simulink model "SF049A_LoaMgr"  (R2013b)
settings: Solver=FixedStepDiscrete  SolverMode=SingleTasking  StartTime=0.0  StopTime=1  FixedStep=0.002  RelTol=1e-3
undefined symbols (not defined in the file): CURRMEASLOAMTGTNMASK_CNT_U08, IVTRLOAMTGTNMASK_CNT_U08, LoaCtrldShtdwn, LoaCurrMeasIdptSigNrFlt, LoaHwTqIdptSigNrFlt, LoaImdtShtdwn, LoaIvtrIdptSigNrFlt, LOAMAXSLEW_ULSPERSEC_F32, LoaMgrCurrIvtrMtgtnRate, LoaMgrCurrIvtrMtgtnSca, LoaMgrCurrIvtrMtgtnScaZeroEna, LoaMgrCurrMeasIdptSig0Resp, LoaMgrCurrMeasIdptSig1Resp, LoaMgrCurrMeasIdptSig2Resp, LoaMgrCurrMeasIdptSigFltThd, LoaMgrCurrMeasMtgtnRate, LoaMgrCurrMeasMtgtnSca, LoaMgrCurrMeasMtgtnScaZeroEna, LoaMgrFadeOutStRate, LoaMgrHwTqIdptSig0NoTqLoaResp, LoaMgrHwTqIdptSig1NoTqLoaResp, LoaMgrHwTqIdptSig2Resp, LoaMgrHwTqIdptSig4Resp, LoaMgrHwTqIdptSigFltThd, LoaMgrHwTqLoaAvlResp, LoaMgrIvtrIdptSig0Resp, LoaMgrIvtrIdptSig1Resp, LoaMgrIvtrIdptSig2Resp, LoaMgrIvtrIdptSigFltThd, LoaMgrIvtrMtgtnRate, LoaMgrIvtrMtgtnSca, LoaMgrIvtrMtgtnScaZeroEna, LoaMgrLimdStRate, LoaMgrLimdStSca, LoaMgrMotAgAvlSnsrlsResp, LoaMgrMotAgIdptSig0NoSnsrlsResp, LoaMgrMotAgIdptSig1NoSnsrlsResp, LoaMgrMotAgIdptSig2Resp, LoaMgrMotAgIdptSig3Resp, LoaMgrMotAgIdptSigFltThd, LoaMgrMotAgMtgtnRate, LoaMgrMotAgMtgtnSca, LoaMgrMotAgMtgtnScaZeroEna, LoaMotAgIdptSigNrFlt, LOASCAONE_ULS_F32, LOASCAZERO_ULS_F32, LoaSt1, LOASTIMDTSHTDWN_CNT_U08, LOASTNORM_CNT_U08, LOASTSWMTGTN_CNT_U08, MAXCURRMEASIDPTSIGALLWD_CNT_U08, MAXHWTQIDPTSIGALLWD_CNT_U08, MAXIVTRIDPTSIGALLWD_CNT_U08, MAXMOTAGMECLIDPTSIGALLWD_CNT_U08, NODEBSTEP_CNT_U16, NtcSts1, SigQlfr1
libraries: simulink x30, NxtrMin x4, NxtrMax x4, NxtrLim x2
(part 2 of 7)

== system SF049A_LoaMgr/ISO Fault Debounce/DiagMgr/NTCSTS_PREFAILD ==
  EA : Inport
  DS : Inport  Port=2
  TS : Inport  Port=3
  Qlf : Inport  Port=4
  Action Port : ActionPort  ActionType=case
  CopyRight2 : Subsystem  Description=|  mask(Copyright Information){none=on}
      | Copyright info block.                                               
      |                                                                     
      | Place copyright information at the top of every subsystem in design.
      mask prompts: none "No parameters"
      mask help: Place copyright information at the top of every subsystem in design.
      mask Display:
      | NxtrConf = 'Nexteer Confidential';
      | 
      | sys = bdroot; %handle for the current model ("system")
      | first = get_param(sys,'Created');
      | first = first(end-3:end);  %year is last four digits
      | 
      | last = get_param(sys,'LastModifiedDate');
      | if isempty(last)
      |     last = datestr(now,'yyyy');
      | else
      |     last = last(end-3:end);
      | end
      | 
      | if strcmp(first,last)
      |     fprintf('%s -- Copyright %s Nexteer',NxtrConf,first)
      | else
      |     fprintf('%s -- %s%s- %s Nexteer',NxtrConf,char(169),first,last)
      | end
  Data Type Conversion : DataTypeConversion
  If : If  IfExpression=u1 <= 0
  If Action Subsystem : Subsystem  TreatAsAtomicUnit=on
  If Action Subsystem1 : Subsystem  TreatAsAtomicUnit=on
  Merge : Merge
  Merge1 : Merge
  EAo : Outport
  Qlfo : Outport  Port=2
  wires:
  EA/1 -> If Action Subsystem1/2(EA), If/1
  If/1 -> If Action Subsystem/Action
  If/2 -> If Action Subsystem1/Action
  DS/1 -> Data Type Conversion/1, If Action Subsystem1/1(DS)
  TS/1 -> If Action Subsystem1/4(TS)
  If Action Subsystem/1(EAo) -> Merge/1
  If Action Subsystem1/1(EAo) -> Merge/2
  If Action Subsystem1/2(Qlfo) -> Merge1/2
  If Action Subsystem/2(Qlfo) -> Merge1/1
  Merge/1 -> EAo/1
  Merge1/1 -> Qlfo/1
  Qlf/1 -> If Action Subsystem/2(Qlf), If Action Subsystem1/3(Qlf)
  Data Type Conversion/1 -> If Action Subsystem/1(DS)

== system SF049A_LoaMgr/ISO Fault Debounce/DiagMgr/NTCSTS_PREPASSD ==
  EA : Inport
  DS : Inport  Port=2
  TS : Inport  Port=3
  Qlf : Inport  Port=4
  Action Port : ActionPort  ActionType=case
  CopyRight2 : Subsystem  Description=|  mask(Copyright Information){none=on}
      | Copyright info block.                                               
      |                                                                     
      | Place copyright information at the top of every subsystem in design.
      mask prompts: none "No parameters"
      mask help: Place copyright information at the top of every subsystem in design.
      mask Display:
      | NxtrConf = 'Nexteer Confidential';
      | 
      | sys = bdroot; %handle for the current model ("system")
      | first = get_param(sys,'Created');
      | first = first(end-3:end);  %year is last four digits
      | 
      | last = get_param(sys,'LastModifiedDate');
      | if isempty(last)
      |     last = datestr(now,'yyyy');
      | else
      |     last = last(end-3:end);
      | end
      | 
      | if strcmp(first,last)
      |     fprintf('%s -- Copyright %s Nexteer',NxtrConf,first)
      | else
      |     fprintf('%s -- %s%s- %s Nexteer',NxtrConf,char(169),first,last)
      | end
  If : If  NumInputs=2  IfExpression=u1 <= u2
  If Action Subsystem : Subsystem  TreatAsAtomicUnit=on
  If Action Subsystem1 : Subsystem  TreatAsAtomicUnit=on
  Merge : Merge
  Merge1 : Merge
  QlfPassd : Constant  Value=SigQlfr1.SIGQLFR_PASSD  OutDataTypeStr=Enum: SigQlfr1
  Sum : Sum  Inputs=|+-
  Unary Minus : UnaryMinus
  EAo : Outport
  Qlfo : Outport  Port=2
  wires:
  EA/1 -> Sum/1
  DS/1 -> Sum/2
  Sum/1 -> If Action Subsystem1/1(In1), If/1
  TS/1 -> [Threshold], If/2
  If/1 -> If Action Subsystem/Action
  Unary Minus/1 -> If Action Subsystem/1(In1)
  If Action Subsystem/1(Out1) -> Merge/1
  If Action Subsystem1/1(Out1) -> Merge/2
  Merge/1 -> EAo/1
  If Action Subsystem/2(Out2) -> Merge1/1
  If Action Subsystem1/2(Out2) -> Merge1/2
  Merge1/1 -> Qlfo/1
  QlfPassd/1 -> If Action Subsystem/2(In2)
  Qlf/1 -> If Action Subsystem1/2(In2)
  If/2 -> If Action Subsystem1/Action
  [Threshold] -> Unary Minus/1

== system SF049A_LoaMgr/ISO Fault Debounce/DiagMgr/Set Latch ==
  In1 : Inport
  Action Port : ActionPort  ActionType=then
  Out1 : Outport
  wires:
  In1/1 -> Out1/1

== system SF049A_LoaMgr/LoaMgr/LoaMgrInit1/CopyRight2 ==

== system SF049A_LoaMgr/LoaMgr/LoaMgrInit1/NTC_Fault1 ==
  NtcNr : Inport
  NtcStInfo : Inport  Port=2
  NtcSts : Inport  Port=3
  DebStep : Inport  Port=4
  SetNtcSts : Subsystem  RequirementInfo={} %GIDa_2d4748e1_3eff_489d_bd26_29790f45e4ce  TreatAsAtomicUnit=on
      settings: RTWSystemCode=Inline
  wires:
  NtcStInfo/1 -> SetNtcSts/2(NtcStInfo)
  DebStep/1 -> SetNtcSts/4(DebStep)
  NtcSts/1 -> SetNtcSts/3(NtcSts)
  NtcNr/1 -> SetNtcSts/1(NtcNr)  "NtcNr"

== system SF049A_LoaMgr/LoaMgr/LoaMgrInit1/NTC_Fault2 ==
  NtcNr : Inport
  NtcStInfo : Inport  Port=2
  NtcSts : Inport  Port=3
  DebStep : Inport  Port=4
  SetNtcSts : Subsystem  RequirementInfo={} %GIDa_343ebabd_6576_496c_8444_ca2dd1733188  TreatAsAtomicUnit=on
      settings: RTWSystemCode=Inline
  wires:
  NtcNr/1 -> SetNtcSts/1(NtcNr)  "NtcNr"
  NtcSts/1 -> SetNtcSts/3(NtcSts)
  DebStep/1 -> SetNtcSts/4(DebStep)
  NtcStInfo/1 -> SetNtcSts/2(NtcStInfo)

== system SF049A_LoaMgr/LoaMgr/LoaMgrInit1/NTC_Fault3 ==
  NtcNr : Inport
  NtcStInfo : Inport  Port=2
  NtcSts : Inport  Port=3
  DebStep : Inport  Port=4
  SetNtcSts : Subsystem  RequirementInfo={} %GIDa_1c324736_f34f_4c75_bc42_99b95d6fd5a4  TreatAsAtomicUnit=on
      settings: RTWSystemCode=Inline
  wires:
  NtcNr/1 -> SetNtcSts/1(NtcNr)  "NtcNr"
  NtcSts/1 -> SetNtcSts/3(NtcSts)
  DebStep/1 -> SetNtcSts/4(DebStep)
  NtcStInfo/1 -> SetNtcSts/2(NtcStInfo)

== system SF049A_LoaMgr/LoaMgr/LoaMgrInit1/NTC_Fault4 ==
  NtcNr : Inport
  NtcStInfo : Inport  Port=2
  NtcSts : Inport  Port=3
  DebStep : Inport  Port=4
  SetNtcSts : Subsystem  RequirementInfo={} %GIDa_54e2fc55_0d47_4369_9e98_1a1b99df313d  TreatAsAtomicUnit=on
      settings: RTWSystemCode=Inline
  wires:
  NtcStInfo/1 -> SetNtcSts/2(NtcStInfo)
  DebStep/1 -> SetNtcSts/4(DebStep)
  NtcSts/1 -> SetNtcSts/3(NtcSts)
  NtcNr/1 -> SetNtcSts/1(NtcNr)  "NtcNr"

== system SF049A_LoaMgr/LoaMgr/LoaMgrInit1/NTC_Fault5 ==
  NtcNr : Inport
  NtcStInfo : Inport  Port=2
  NtcSts : Inport  Port=3
  DebStep : Inport  Port=4
  SetNtcSts : Subsystem  RequirementInfo={} %GIDa_03bf9754_a4f9_470a_8d26_b2877fc3dca8  TreatAsAtomicUnit=on
      settings: RTWSystemCode=Inline
  wires:
  NtcNr/1 -> SetNtcSts/1(NtcNr)  "NtcNr"
  NtcSts/1 -> SetNtcSts/3(NtcSts)
  DebStep/1 -> SetNtcSts/4(DebStep)
  NtcStInfo/1 -> SetNtcSts/2(NtcStInfo)

== system SF049A_LoaMgr/LoaMgr/LoaMgrInit1/NTC_Fault6 ==
  NtcNr : Inport
  NtcStInfo : Inport  Port=2
  NtcSts : Inport  Port=3
  DebStep : Inport  Port=4
  SetNtcSts : Subsystem  RequirementInfo={} %GIDa_5a3bfc9a_be7c_4214_b245_692942f94cc7  TreatAsAtomicUnit=on
      settings: RTWSystemCode=Inline
  wires:
  NtcNr/1 -> SetNtcSts/1(NtcNr)  "NtcNr"
  NtcSts/1 -> SetNtcSts/3(NtcSts)
  DebStep/1 -> SetNtcSts/4(DebStep)
  NtcStInfo/1 -> SetNtcSts/2(NtcStInfo)

== system SF049A_LoaMgr/LoaMgr/LoaMgrPer1/Arbitrate_Responses ==
  note: Individual responses can set boolean flags to true to direct downstream functions.
      | The combination of individual responses generates its own "multiple mitigation response".
      | The final LoaState response will be the worst case of individual and "multiple mitigation" responses.
  RespMux : Inport
  CntSwBasdMtgtn : Subsystem
  CopyRight2 : Subsystem  Description=|  mask(Copyright Information){none=on}
      | Copyright info block.                                               
      |                                                                     
      | Place copyright information at the top of every subsystem in design.
      mask prompts: none "No parameters"
      mask help: Place copyright information at the top of every subsystem in design.
      mask Display:
      | NxtrConf = 'Nexteer Confidential';
      | 
      | sys = bdroot; %handle for the current model ("system")
      | first = get_param(sys,'Created');
      | first = first(end-3:end);  %year is last four digits
      | 
      | last = get_param(sys,'LastModifiedDate');
      | if isempty(last)
      |     last = datestr(now,'yyyy');
      | else
      |     last = last(end-3:end);
      | end
      | 
      | if strcmp(first,last)
      |     fprintf('%s -- Copyright %s Nexteer',NxtrConf,first)
      | else
      |     fprintf('%s -- %s%s- %s Nexteer',NxtrConf,char(169),first,last)
      | end
  Demux : Demux
  Demux1 : Demux
  Mux : Mux
  SelFinalResp : Subsystem
  LoaState : Outport  RequirementInfo={} %GIDa_5b4aaf8e_36d6_468e_97c1_31f6ab28a5ed
  SwMtgtnEnMux : Outport  Port=2
  wires:
  SelFinalResp/1(LoaSt) -> LoaState/1
  Demux1/4 -> SelFinalResp/5(IvtrResp)
  Demux1/3 -> SelFinalResp/4(CurrMeasResp)
  Demux1/2 -> SelFinalResp/3(MotAgResp)
  Demux1/1 -> SelFinalResp/2(HwTqResp)
  RespMux/1 -> Demux/1, Demux1/1
  CntSwBasdMtgtn/5(MultiMtgtnResp) -> SelFinalResp/1(MultiMtgtnResp)
  Mux/1 -> SwMtgtnEnMux/1
  CntSwBasdMtgtn/4(IvtrLoaMtgtnEna) -> Mux/4  "IvtrLoaMtgtnEna"
  CntSwBasdMtgtn/3(CurrMeasLoaMtgtnEna) -> Mux/3  "CurrMeasLoaMtgtnEna"
  CntSwBasdMtgtn/2(MotAgLoaMtgtnEna) -> Mux/2  "MotAgLoaMtgtnEna"
  CntSwBasdMtgtn/1(HwTqLoaMtgtnEna) -> Mux/1  "HwTqLoaMtgtnEna"
  Demux/4 -> CntSwBasdMtgtn/4(IvtrResp)
  Demux/3 -> CntSwBasdMtgtn/3(CurrMeasResp)
  Demux/2 -> CntSwBasdMtgtn/2(MotAgResp)
  Demux/1 -> CntSwBasdMtgtn/1(HwTqResp)

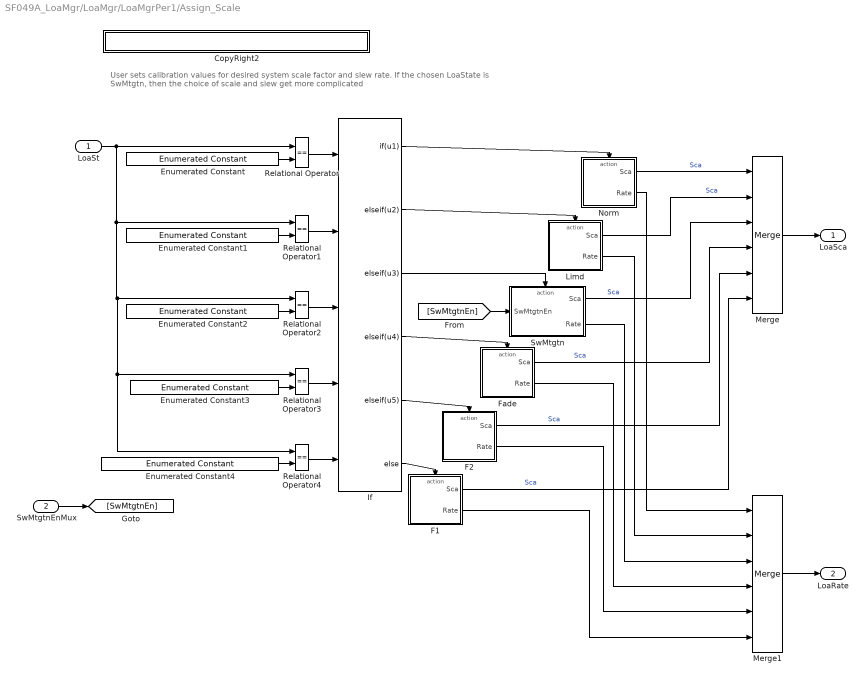
== system SF049A_LoaMgr/LoaMgr/LoaMgrPer1/Assign_Scale ==
  note: User sets calibration values for desired system scale factor and slew rate.  If the chosen LoaState is SwMtgtn, then the choice of
      | scale and slew get more complicated
  LoaSt : Inport  RequirementInfo={} %GIDa_be3f296e_dcfd_40f3_bb44_9f6a3a049e3e
  SwMtgtnEnMux : Inport  RequirementInfo={} %GIDa_b523e120_0d97_4e71_b546_a709c6101313  Port=2
  CopyRight2 : Subsystem  Description=|  mask(Copyright Information){none=on}
      | Copyright info block.                                               
      |                                                                     
      | Place copyright information at the top of every subsystem in design.
      mask prompts: none "No parameters"
      mask help: Place copyright information at the top of every subsystem in design.
      mask Display:
      | NxtrConf = 'Nexteer Confidential';
      | 
      | sys = bdroot; %handle for the current model ("system")
      | first = get_param(sys,'Created');
      | first = first(end-3:end);  %year is last four digits
      | 
      | last = get_param(sys,'LastModifiedDate');
      | if isempty(last)
      |     last = datestr(now,'yyyy');
      | else
      |     last = last(end-3:end);
      | end
      | 
      | if strcmp(first,last)
      |     fprintf('%s -- Copyright %s Nexteer',NxtrConf,first)
      | else
      |     fprintf('%s -- %s%s- %s Nexteer',NxtrConf,char(169),first,last)
      | end
  Enumerated Constant : simulink/Sources/Enumerated Constant  RequirementInfo="{'linktype_rmi_doors' '00012fd5 (/E-STEER Core/SubSystem Specifications/Application Functions - EA4/SF049A Loss of Assist Manager)' '#SF049A_148' 'true' 'REQ:  SF049A_148' '' } %GIDa_17825fe3_cb07_42dd_b86d_f0b5a1a9354d"  OutDataTypeStr=Enum: LoaSt1  Value=LoaSt1.LOAST_NORM  SampleTime=inf
  Enumerated Constant1 : simulink/Sources/Enumerated Constant  RequirementInfo="{'linktype_rmi_doors' '00012fd5 (/E-STEER Core/SubSystem Specifications/Application Functions - EA4/SF049A Loss of Assist Manager)' '#SF049A_149' 'true' 'REQ:  SF049A_149' '' } %GIDa_cfc06f6d_46aa_46c6_9fa9_eb7ac3338082"  OutDataTypeStr=Enum: LoaSt1  Value=LoaSt1.LOAST_LIMD  SampleTime=inf
  Enumerated Constant2 : simulink/Sources/Enumerated Constant  RequirementInfo={} %GIDa_ef22ac21_1988_4c68_a743_2324f025e450  OutDataTypeStr=Enum: LoaSt1  Value=LoaSt1.LOAST_SWBASDMTGTN  SampleTime=inf
  Enumerated Constant3 : simulink/Sources/Enumerated Constant  RequirementInfo="{'linktype_rmi_doors' '00012fd5 (/E-STEER Core/SubSystem Specifications/Application Functions - EA4/SF049A Loss of Assist Manager)' '#SF049A_150' 'true' 'REQ:  SF049A_150' '' } %GIDa_f981875f_77ac_4a28_a7ae_f689b0863588"  OutDataTypeStr=Enum: LoaSt1  Value=LoaSt1.LOAST_FADEOUT  SampleTime=inf
  Enumerated Constant4 : simulink/Sources/Enumerated Constant  RequirementInfo="{'linktype_rmi_doors' '00012fd5 (/E-STEER Core/SubSystem Specifications/Application Functions - EA4/SF049A Loss of Assist Manager)' '#SF049A_151' 'true' 'REQ:  SF049A_151' '' } %GIDa_3c24a642_0c96_4a97_ac7e_bcddbe438dc4"  OutDataTypeStr=Enum: LoaSt1  Value=LoaSt1.LOAST_CTRLDSHTDWNREQD  SampleTime=inf
  F1 : Subsystem  RequirementInfo="{'linktype_rmi_doors' '00012fd5 (/E-STEER Core/SubSystem Specifications/Application Functions - EA4/SF049A Loss of Assist Manager)' '#SF049A_152' 'true' 'REQ:  SF049A_152' '' } %GIDa_bd57649e_89e1_4cc3_9888_fae0c4de09d1"  TreatAsAtomicUnit=on
      settings: RTWSystemCode=Inline
  F2 : Subsystem  RequirementInfo="{'linktype_rmi_doors' '00012fd5 (/E-STEER Core/SubSystem Specifications/Application Functions - EA4/SF049A Loss of Assist Manager)' '#SF049A_151' 'true' 'REQ:  SF049A_151' '' } %GIDa_610c1087_6c21_4097_a9b8_f7e698a4c3a1"  TreatAsAtomicUnit=on
      settings: RTWSystemCode=Inline
  Fade : Subsystem  RequirementInfo="{'linktype_rmi_doors' '00012fd5 (/E-STEER Core/SubSystem Specifications/Application Functions - EA4/SF049A Loss of Assist Manager)' '#SF049A_150' 'true' 'REQ:  SF049A_150' '' } %GIDa_fcbfa092_767e_495f_8177_f4025c07d9b8"  TreatAsAtomicUnit=on
      settings: RTWSystemCode=Inline
  If : If  RequirementInfo="{'linktype_rmi_doors' '00012fd5 (/E-STEER Core/SubSystem Specifications/Application Functions - EA4/SF049A Loss of Assist Manager)' '#SF049A_148' 'true' 'REQ:  SF049A_148' '' ; 'linktype_rmi_doors' '00012fd5 (/E-STEER Core/SubSystem Specifications/Application Functions - EA4/SF049A Loss of Assist Manager)' '#SF049A_149' 'true' 'REQ:  SF049A_149' '' ; 'linktype_rmi_doors' '00012fd5 (/E-STEER Core/SubSystem Specifications/Application Functions - EA4/SF049A Loss of Assist Manager)' '#SF049A_150' 'true' 'REQ:  SF049A_150' '' ; 'linktype_rmi_doors' '00012fd5 (/E-STEER Core/SubSystem Specifications/Application Functions - EA4/SF049A Loss of Assist Manager)' '#SF049A_151' 'true' 'REQ:  SF049A_151' '' ; 'linktype_rmi_doors' '00012fd5 (/E-STEER Core/SubSystem Specifications/Application Functions - EA4/SF049A Loss of Assist Manager)' '#SF049A_152' 'true' 'REQ:  SF049A_152' '' } %GIDa_9a1115ea_d572_4d7a_85a3_b7a7c80caa4b"  NumInputs=5  IfExpression=u1  ElseIfExpressions=u2, u3,u4,u5
  Limd : Subsystem  RequirementInfo="{'linktype_rmi_doors' '00012fd5 (/E-STEER Core/SubSystem Specifications/Application Functions - EA4/SF049A Loss of Assist Manager)' '#SF049A_149' 'true' 'REQ:  SF049A_149' '' } %GIDa_75ef6631_0859_46ba_a6af_57943735bc8c"  TreatAsAtomicUnit=on
      settings: RTWSystemCode=Inline
  Merge : Merge  RequirementInfo="{'linktype_rmi_doors' '00012fd5 (/E-STEER Core/SubSystem Specifications/Application Functions - EA4/SF049A Loss of Assist Manager)' '#SF049A_148' 'true' 'REQ:  SF049A_148' '' ; 'linktype_rmi_doors' '00012fd5 (/E-STEER Core/SubSystem Specifications/Application Functions - EA4/SF049A Loss of Assist Manager)' '#SF049A_149' 'true' 'REQ:  SF049A_149' '' ; 'linktype_rmi_doors' '00012fd5 (/E-STEER Core/SubSystem Specifications/Application Functions - EA4/SF049A Loss of Assist Manager)' '#SF049A_150' 'true' 'REQ:  SF049A_150' '' ; 'linktype_rmi_doors' '00012fd5 (/E-STEER Core/SubSystem Specifications/Application Functions - EA4/SF049A Loss of Assist Manager)' '#SF049A_151' 'true' 'REQ:  SF049A_151' '' ; 'linktype_rmi_doors' '00012fd5 (/E-STEER Core/SubSystem Specifications/Application Functions - EA4/SF049A Loss of Assist Manager)' '#SF049A_152' 'true' 'REQ:  SF049A_152' '' } %GIDa_063df2a1_507e_4f47_9f63_ed3c525ef632"  Inputs=6
  Merge1 : Merge  RequirementInfo="{'linktype_rmi_doors' '00012fd5 (/E-STEER Core/SubSystem Specifications/Application Functions - EA4/SF049A Loss of Assist Manager)' '#SF049A_148' 'true' 'REQ:  SF049A_148' '' ; 'linktype_rmi_doors' '00012fd5 (/E-STEER Core/SubSystem Specifications/Application Functions - EA4/SF049A Loss of Assist Manager)' '#SF049A_149' 'true' 'REQ:  SF049A_149' '' ; 'linktype_rmi_doors' '00012fd5 (/E-STEER Core/SubSystem Specifications/Application Functions - EA4/SF049A Loss of Assist Manager)' '#SF049A_150' 'true' 'REQ:  SF049A_150' '' ; 'linktype_rmi_doors' '00012fd5 (/E-STEER Core/SubSystem Specifications/Application Functions - EA4/SF049A Loss of Assist Manager)' '#SF049A_151' 'true' 'REQ:  SF049A_151' '' ; 'linktype_rmi_doors' '00012fd5 (/E-STEER Core/SubSystem Specifications/Application Functions - EA4/SF049A Loss of Assist Manager)' '#SF049A_152' 'true' 'REQ:  SF049A_152' '' } %GIDa_9f0103d2_b2d4_4579_bb1c_e06b6977214b"  Inputs=6
  Norm : Subsystem  RequirementInfo="{'linktype_rmi_doors' '00012fd5 (/E-STEER Core/SubSystem Specifications/Application Functions - EA4/SF049A Loss of Assist Manager)' '#SF049A_148' 'true' 'REQ:  SF049A_148' '' } %GIDa_2363d845_a935_4fe8_afb6_f6c17a6fc808"  TreatAsAtomicUnit=on
      settings: RTWSystemCode=Inline
  Relational Operator : RelationalOperator  RequirementInfo="{'linktype_rmi_doors' '00012fd5 (/E-STEER Core/SubSystem Specifications/Application Functions - EA4/SF049A Loss of Assist Manager)' '#SF049A_148' 'true' 'REQ:  SF049A_148' '' } %GIDa_095c9634_e6ee_4ed8_bb0d_0a1cb03bc836"  Operator===  OutDataTypeStr=boolean
  Relational Operator1 : RelationalOperator  RequirementInfo="{'linktype_rmi_doors' '00012fd5 (/E-STEER Core/SubSystem Specifications/Application Functions - EA4/SF049A Loss of Assist Manager)' '#SF049A_149' 'true' 'REQ:  SF049A_149' '' } %GIDa_353a2502_0a9f_48b7_9fef_cec66dc0707c"  Operator===  OutDataTypeStr=boolean
  Relational Operator2 : RelationalOperator  RequirementInfo={} %GIDa_a6472754_471f_43b6_8ccc_293474aaeb6f  Operator===  OutDataTypeStr=boolean
  Relational Operator3 : RelationalOperator  RequirementInfo="{'linktype_rmi_doors' '00012fd5 (/E-STEER Core/SubSystem Specifications/Application Functions - EA4/SF049A Loss of Assist Manager)' '#SF049A_150' 'true' 'REQ:  SF049A_150' '' } %GIDa_1cafa691_935b_4f52_ad1f_1a8b7e8d3199"  Operator===  OutDataTypeStr=boolean
  Relational Operator4 : RelationalOperator  RequirementInfo="{'linktype_rmi_doors' '00012fd5 (/E-STEER Core/SubSystem Specifications/Application Functions - EA4/SF049A Loss of Assist Manager)' '#SF049A_151' 'true' 'REQ:  SF049A_151' '' } %GIDa_4980d6ce_f1f3_4944_a48b_75077fb3a6e6"  Operator===  OutDataTypeStr=boolean
  SwMtgtn : Subsystem  RequirementInfo={} %GIDa_2ba28934_9dad_4dc2_b171_77dd04a05cd7  TreatAsAtomicUnit=on
      settings: RTWSystemCode=Inline
  LoaSca : Outport  RequirementInfo={} %GIDa_567a72cb_eb9d_48ca_918a_ed43dbfb5856
  LoaRate : Outport  RequirementInfo={} %GIDa_4b377c46_469c_400c_ba1b_1f854315ac6b  Port=2
  wires:
  SwMtgtn/2(Rate) -> Merge1/3
  SwMtgtn/1(Sca) -> Merge/3  "Sca"
  [SwMtgtnEn] -> SwMtgtn/1(SwMtgtnEn)
  SwMtgtnEnMux/1 -> [SwMtgtnEn]
  Merge1/1 -> LoaRate/1
  F1/2(Rate) -> Merge1/6
  F2/2(Rate) -> Merge1/5
  Fade/2(Rate) -> Merge1/4
  Limd/2(Rate) -> Merge1/2
  Norm/2(Rate) -> Merge1/1
  Merge/1 -> LoaSca/1
  F1/1(Sca) -> Merge/6  "Sca"
  F2/1(Sca) -> Merge/5  "Sca"
  Fade/1(Sca) -> Merge/4  "Sca"
  Limd/1(Sca) -> Merge/2  "Sca"
  Norm/1(Sca) -> Merge/1  "Sca"
  If/6 -> F1/Action
  If/5 -> F2/Action
  If/4 -> Fade/Action
  If/3 -> SwMtgtn/Action
  If/2 -> Limd/Action
  If/1 -> Norm/Action
  Relational Operator4/1 -> If/5
  Relational Operator3/1 -> If/4
  Relational Operator2/1 -> If/3
  Relational Operator1/1 -> If/2
  Relational Operator/1 -> If/1
  Enumerated Constant4/1 -> Relational Operator4/2
  LoaSt/1 -> Relational Operator/1, Relational Operator1/1, Relational Operator2/1, Relational Operator3/1, Relational Operator4/1
  Enumerated Constant3/1 -> Relational Operator3/2
  Enumerated Constant2/1 -> Relational Operator2/2
  Enumerated Constant1/1 -> Relational Operator1/2
  Enumerated Constant/1 -> Relational Operator/2

== system SF049A_LoaMgr/LoaMgr/LoaMgrPer1/Calc_Ivtr_State ==
  note: Nexter coding standards prevent the casting of boolean signals to other datatypes.
      | If that rule did not exist, this logic would use convert blocks to cast each boolean
      | to uint8, then add them up.
  Ivtr1Inactv : Inport  RequirementInfo={} %GIDa_17ac93f8_d6a9_43a2_82a0_7d4f023bfceb
  Ivtr2Inactv : Inport  RequirementInfo={} %GIDa_2d28aecd_eb1d_45c7_985c_cceb95458058  Port=2
  " " : Merge  RequirementInfo="{'linktype_rmi_doors' '00012fd5 (/E-STEER Core/SubSystem Specifications/Application Functions - EA4/SF049A Loss of Assist Manager)' '#SF049A_109' 'true' 'REQ:  SF049A_109' '' } %GIDa_8c4eec8b_af54_40d7_8cac_4715333782d3"
  " 1" : Merge  RequirementInfo="{'linktype_rmi_doors' '00012fd5 (/E-STEER Core/SubSystem Specifications/Application Functions - EA4/SF049A Loss of Assist Manager)' '#SF049A_109' 'true' 'REQ:  SF049A_109' '' } %GIDa_fa6d2c6b_877b_417b_b944_867b75e43a03"
  Add1 : Sum  RequirementInfo="{'linktype_rmi_doors' '00012fd5 (/E-STEER Core/SubSystem Specifications/Application Functions - EA4/SF049A Loss of Assist Manager)' '#SF049A_109' 'true' 'REQ:  SF049A_109' '' } %GIDa_d9a5bc75_1226_4711_9930_dc54fbf2ce48"
  Constant1 : Constant  RequirementInfo="{'linktype_rmi_doors' '00012fd5 (/E-STEER Core/SubSystem Specifications/Application Functions - EA4/SF049A Loss of Assist Manager)' '#SF049A_109' 'true' 'REQ:  SF049A_109' '' } %GIDa_f2ffa765_eea1_4726_ad80_e9135f5bab64"  OutDataTypeStr=uint8
      settings: AttributesFormatString=%<OutDataTypeStr>
  Constant2 : Constant  RequirementInfo="{'linktype_rmi_doors' '00012fd5 (/E-STEER Core/SubSystem Specifications/Application Functions - EA4/SF049A Loss of Assist Manager)' '#SF049A_109' 'true' 'REQ:  SF049A_109' '' } %GIDa_c01fa7dc_7e07_4040_a864_7d5fc01689d3"  Value=0  OutDataTypeStr=uint8
      settings: AttributesFormatString=%<OutDataTypeStr>
  Constant4 : Constant  RequirementInfo="{'linktype_rmi_doors' '00012fd5 (/E-STEER Core/SubSystem Specifications/Application Functions - EA4/SF049A Loss of Assist Manager)' '#SF049A_109' 'true' 'REQ:  SF049A_109' '' } %GIDa_c066b0f6_743d_44d6_a8d4_39d9792cd5a4"  Value=0  OutDataTypeStr=uint8
      settings: AttributesFormatString=%<OutDataTypeStr>
  Constant6 : Constant  RequirementInfo="{'linktype_rmi_doors' '00012fd5 (/E-STEER Core/SubSystem Specifications/Application Functions - EA4/SF049A Loss of Assist Manager)' '#SF049A_109' 'true' 'REQ:  SF049A_109' '' } %GIDa_8c9531b5_421c_4d2b_a54d_10f7a909c9c8"  OutDataTypeStr=uint8
      settings: AttributesFormatString=%<OutDataTypeStr>
  CopyRight2 : Subsystem  Description=|  mask(Copyright Information){none=on}
      | Copyright info block.                                               
      |                                                                     
      | Place copyright information at the top of every subsystem in design.
      mask prompts: none "No parameters"
      mask help: Place copyright information at the top of every subsystem in design.
      mask Display:
      | NxtrConf = 'Nexteer Confidential';
      | 
      | sys = bdroot; %handle for the current model ("system")
      | first = get_param(sys,'Created');
      | first = first(end-3:end);  %year is last four digits
      | 
      | last = get_param(sys,'LastModifiedDate');
      | if isempty(last)
      |     last = datestr(now,'yyyy');
      | else
      |     last = last(end-3:end);
      | end
      | 
      | if strcmp(first,last)
      |     fprintf('%s -- Copyright %s Nexteer',NxtrConf,first)
      | else
      |     fprintf('%s -- %s%s- %s Nexteer',NxtrConf,char(169),first,last)
      | end
  Ivtr1Inactv_IF : If  RequirementInfo="{'linktype_rmi_doors' '00012fd5 (/E-STEER Core/SubSystem Specifications/Application Functions - EA4/SF049A Loss of Assist Manager)' '#SF049A_109' 'true' 'REQ:  SF049A_109' '' } %GIDa_ad9c1b53_37da_4fd2_b63d_bf04c9aae89e"  IfExpression=u1
  Ivtr1Sts_ELSE : Subsystem  RequirementInfo="{'linktype_rmi_doors' '00012fd5 (/E-STEER Core/SubSystem Specifications/Application Functions - EA4/SF049A Loss of Assist Manager)' '#SF049A_109' 'true' 'REQ:  SF049A_109' '' } %GIDa_bcb94737_b9df_4ed2_af66_9c7176aae729"  TreatAsAtomicUnit=on
      settings: RTWSystemCode=Inline
  Ivtr1Sts_THEN : Subsystem  RequirementInfo="{'linktype_rmi_doors' '00012fd5 (/E-STEER Core/SubSystem Specifications/Application Functions - EA4/SF049A Loss of Assist Manager)' '#SF049A_109' 'true' 'REQ:  SF049A_109' '' } %GIDa_41cd9936_3a28_4904_8098_7dae13fd8a93"  TreatAsAtomicUnit=on
      settings: RTWSystemCode=Inline
  Ivtr2Inactv_IF : If  RequirementInfo="{'linktype_rmi_doors' '00012fd5 (/E-STEER Core/SubSystem Specifications/Application Functions - EA4/SF049A Loss of Assist Manager)' '#SF049A_109' 'true' 'REQ:  SF049A_109' '' } %GIDa_404c2653_fc86_45ff_9ed7_e5ac1f0e5768"  IfExpression=u1
  Ivtr2Sts_ELSE : Subsystem  RequirementInfo="{'linktype_rmi_doors' '00012fd5 (/E-STEER Core/SubSystem Specifications/Application Functions - EA4/SF049A Loss of Assist Manager)' '#SF049A_109' 'true' 'REQ:  SF049A_109' '' } %GIDa_59c6efd0_f783_484c_8c28_3a2ac45d5937"  TreatAsAtomicUnit=on
      settings: RTWSystemCode=Inline
  Ivtr2Sts_THEN : Subsystem  RequirementInfo="{'linktype_rmi_doors' '00012fd5 (/E-STEER Core/SubSystem Specifications/Application Functions - EA4/SF049A Loss of Assist Manager)' '#SF049A_109' 'true' 'REQ:  SF049A_109' '' } %GIDa_8ff3aedd_82f3_4c02_888a_1a97d95ddad5"  TreatAsAtomicUnit=on
      settings: RTWSystemCode=Inline
  IvtrIdptSig : Outport  RequirementInfo={} %GIDa_10b5954b_6612_4aaa_85d3_5668a89d45b3
  wires:
  Add1/1 -> IvtrIdptSig/1
  Ivtr1Sts_THEN/1(Out2) -> " "/1
  Constant4/1 -> Ivtr1Sts_THEN/1(In1)
  Ivtr2Inactv_IF/2 -> Ivtr2Sts_ELSE/Action
  Constant1/1 -> Ivtr2Sts_ELSE/1(In1)
  Ivtr1Inactv/1 -> Ivtr1Inactv_IF/1
  Ivtr1Sts_ELSE/1(Out1) -> " "/2
  Constant6/1 -> Ivtr1Sts_ELSE/1(In1)
  Ivtr1Inactv_IF/1 -> Ivtr1Sts_THEN/Action
  Ivtr1Inactv_IF/2 -> Ivtr1Sts_ELSE/Action
  Ivtr2Inactv/1 -> Ivtr2Inactv_IF/1
  Ivtr2Sts_ELSE/1(Out1) -> " 1"/2
  Ivtr2Sts_THEN/1(Out1) -> " 1"/1
  Constant2/1 -> Ivtr2Sts_THEN/1(In1)
  Ivtr2Inactv_IF/1 -> Ivtr2Sts_THEN/Action
  " 1"/1 -> Add1/2
  " "/1 -> Add1/1

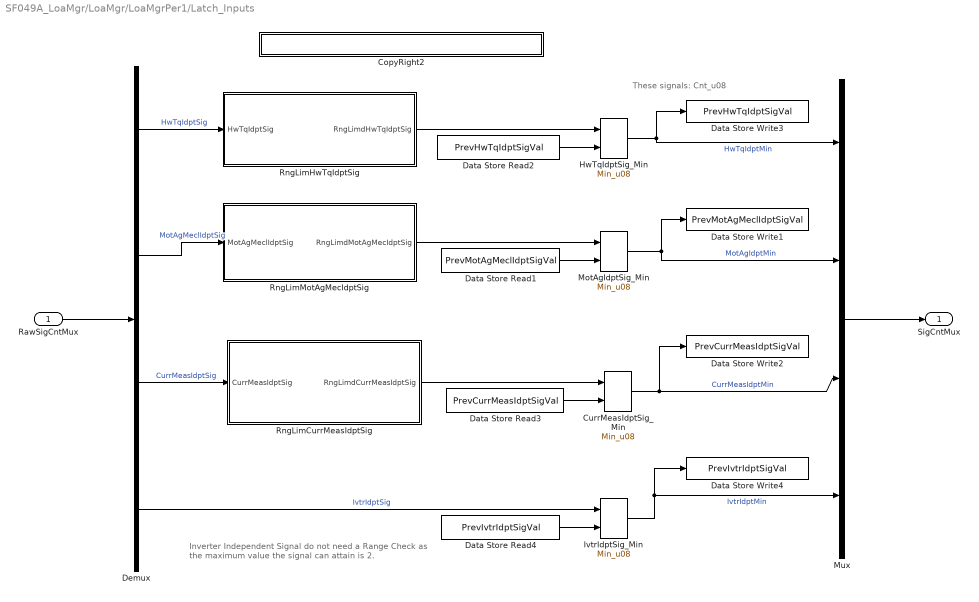
== system SF049A_LoaMgr/LoaMgr/LoaMgrPer1/Latch_Inputs ==
  note: These signals: Cnt_u08
  note: Inverter Independent Signal do not need a Range Check
      | as the maximum value the signal can attain is 2.
  RawSigCntMux : Inport  RequirementInfo={} %GIDa_03401462_221d_4025_a942_72f0becf40a8
  CopyRight2 : Subsystem  Description=|  mask(Copyright Information){none=on}
      | Copyright info block.                                               
      |                                                                     
      | Place copyright information at the top of every subsystem in design.
      mask prompts: none "No parameters"
      mask help: Place copyright information at the top of every subsystem in design.
      mask Display:
      | NxtrConf = 'Nexteer Confidential';
      | 
      | sys = bdroot; %handle for the current model ("system")
      | first = get_param(sys,'Created');
      | first = first(end-3:end);  %year is last four digits
      | 
      | last = get_param(sys,'LastModifiedDate');
      | if isempty(last)
      |     last = datestr(now,'yyyy');
      | else
      |     last = last(end-3:end);
      | end
      | 
      | if strcmp(first,last)
      |     fprintf('%s -- Copyright %s Nexteer',NxtrConf,first)
      | else
      |     fprintf('%s -- %s%s- %s Nexteer',NxtrConf,char(169),first,last)
      | end
  CurrMeasIdptSig_Min : NxtrMin/Min_u08  RequirementInfo="{'linktype_rmi_doors' '00012fd5 (/E-STEER Core/SubSystem Specifications/Application Functions - EA4/SF049A Loss of Assist Manager)' '#SF049A_117' 'true' 'REQ:  SF049A_117' '' } %GIDa_0ce0f2ef_636e_4c54_a36a_8d4724b4e3a7"  SFunctionSpec="uint8 y1 = Min_u08( uint8 u1,  uint8 u2)"  ShowSpec=off
      settings: AttributesFormatString=%<Name>
  Data Store Read1 : DataStoreRead  RequirementInfo="{'linktype_rmi_doors' '00012fd5 (/E-STEER Core/SubSystem Specifications/Application Functions - EA4/SF049A Loss of Assist Manager)' '#SF049A_115' 'true' 'REQ:  SF049A_115' '' } %GIDa_9ae9e2de_08b4_460a_a3d6_d4f3fe289168"  DataStoreName=PrevMotAgMeclIdptSigVal
  Data Store Read2 : DataStoreRead  RequirementInfo="{'linktype_rmi_doors' '00012fd5 (/E-STEER Core/SubSystem Specifications/Application Functions - EA4/SF049A Loss of Assist Manager)' '#SF049A_113' 'true' 'REQ:  SF049A_113' '' } %GIDa_ae546d19_45c8_41b4_bd96_efc0d26e0555"  DataStoreName=PrevHwTqIdptSigVal
  Data Store Read3 : DataStoreRead  RequirementInfo="{'linktype_rmi_doors' '00012fd5 (/E-STEER Core/SubSystem Specifications/Application Functions - EA4/SF049A Loss of Assist Manager)' '#SF049A_117' 'true' 'REQ:  SF049A_117' '' } %GIDa_e17a90c5_6774_4118_af85_392a665a6c8c"  DataStoreName=PrevCurrMeasIdptSigVal
  Data Store Read4 : DataStoreRead  RequirementInfo="{'linktype_rmi_doors' '00012fd5 (/E-STEER Core/SubSystem Specifications/Application Functions - EA4/SF049A Loss of Assist Manager)' '#SF049A_165' 'true' 'REQ:  SF049A_165' '' } %GIDa_9dafc192_a0b1_4bd4_9bad_86056378474a"  DataStoreName=PrevIvtrIdptSigVal
  Data Store Write1 : DataStoreWrite  RequirementInfo="{'linktype_rmi_doors' '00012fd5 (/E-STEER Core/SubSystem Specifications/Application Functions - EA4/SF049A Loss of Assist Manager)' '#SF049A_115' 'true' 'REQ:  SF049A_115' '' } %GIDa_29e9194e_4f8b_4b1d_aea4_eb97ed133575"  DataStoreName=PrevMotAgMeclIdptSigVal
  Data Store Write2 : DataStoreWrite  RequirementInfo="{'linktype_rmi_doors' '00012fd5 (/E-STEER Core/SubSystem Specifications/Application Functions - EA4/SF049A Loss of Assist Manager)' '#SF049A_117' 'true' 'REQ:  SF049A_117' '' } %GIDa_55c38956_b346_427f_ab3a_f81c6a8a0b6c"  DataStoreName=PrevCurrMeasIdptSigVal
  Data Store Write3 : DataStoreWrite  RequirementInfo="{'linktype_rmi_doors' '00012fd5 (/E-STEER Core/SubSystem Specifications/Application Functions - EA4/SF049A Loss of Assist Manager)' '#SF049A_113' 'true' 'REQ:  SF049A_113' '' } %GIDa_b03c1152_84d2_43bc_b770_d2cf60d845c1"  DataStoreName=PrevHwTqIdptSigVal
  Data Store Write4 : DataStoreWrite  RequirementInfo="{'linktype_rmi_doors' '00012fd5 (/E-STEER Core/SubSystem Specifications/Application Functions - EA4/SF049A Loss of Assist Manager)' '#SF049A_165' 'true' 'REQ:  SF049A_165' '' } %GIDa_0c171b76_5e9e_49a9_a60c_9ccb4cddf847"  DataStoreName=PrevIvtrIdptSigVal
  Demux : Demux
  HwTqIdptSig_Min : NxtrMin/Min_u08  RequirementInfo="{'linktype_rmi_doors' '00012fd5 (/E-STEER Core/SubSystem Specifications/Application Functions - EA4/SF049A Loss of Assist Manager)' '#SF049A_113' 'true' 'REQ:  SF049A_113' '' } %GIDa_e902107c_163b_483a_abcd_f0d0557c80c5"  SFunctionSpec="uint8 y1 = Min_u08( uint8 u1,  uint8 u2)"  ShowSpec=off
      settings: AttributesFormatString=%<Name>
  IvtrIdptSig_Min : NxtrMin/Min_u08  RequirementInfo="{'linktype_rmi_doors' '00012fd5 (/E-STEER Core/SubSystem Specifications/Application Functions - EA4/SF049A Loss of Assist Manager)' '#SF049A_165' 'true' 'REQ:  SF049A_165' '' } %GIDa_54ad2cca_3986_4e48_8327_015e36ef6428"  SFunctionSpec="uint8 y1 = Min_u08( uint8 u1,  uint8 u2)"  ShowSpec=off
      settings: AttributesFormatString=%<Name>
  MotAgIdptSig_Min : NxtrMin/Min_u08  RequirementInfo="{'linktype_rmi_doors' '00012fd5 (/E-STEER Core/SubSystem Specifications/Application Functions - EA4/SF049A Loss of Assist Manager)' '#SF049A_115' 'true' 'REQ:  SF049A_115' '' } %GIDa_729108a7_8cea_4925_8ebc_109a82dcda8d"  SFunctionSpec="uint8 y1 = Min_u08( uint8 u1,  uint8 u2)"  ShowSpec=off
      settings: AttributesFormatString=%<Name>
  Mux : Mux
  RngLimCurrMeasIdptSig : Subsystem  RequirementInfo={} %GIDa_17525477_fe37_4595_9c78_5940305cfa6d
  RngLimHwTqIdptSig : Subsystem  RequirementInfo={} %GIDa_f02e1821_ae3d_4c97_9468_40b3ec10f94b
  RngLimMotAgMecIdptSig : Subsystem  RequirementInfo={} %GIDa_2a8a07b8_470b_41a4_ba58_569314191d31
  SigCntMux : Outport  RequirementInfo={} %GIDa_a6a4c245_2884_4e87_a35b_a962781c4fa6
  wires:
  Data Store Read3/1 -> CurrMeasIdptSig_Min/2
  RngLimCurrMeasIdptSig/1(RngLimdCurrMeasIdptSig) -> CurrMeasIdptSig_Min/1
  Data Store Read2/1 -> HwTqIdptSig_Min/2
  Data Store Read4/1 -> IvtrIdptSig_Min/2
  Data Store Read1/1 -> MotAgIdptSig_Min/2
  MotAgIdptSig_Min/1 -> Data Store Write1/1, Mux/2  "MotAgIdptMin"
  RngLimHwTqIdptSig/1(RngLimdHwTqIdptSig) -> HwTqIdptSig_Min/1
  RngLimMotAgMecIdptSig/1(RngLimdMotAgMecIdptSig) -> MotAgIdptSig_Min/1
  Demux/1 -> RngLimHwTqIdptSig/1(HwTqIdptSig)  "HwTqIdptSig"
  RawSigCntMux/1 -> Demux/1
  Mux/1 -> SigCntMux/1
  Demux/3 -> RngLimCurrMeasIdptSig/1(CurrMeasIdptSig)  "CurrMeasIdptSig"
  IvtrIdptSig_Min/1 -> Mux/4, Data Store Write4/1  "IvtrIdptMin"
  Demux/4 -> IvtrIdptSig_Min/1  "IvtrIdptSig"
  CurrMeasIdptSig_Min/1 -> Data Store Write2/1, Mux/3  "CurrMeasIdptMin"
  HwTqIdptSig_Min/1 -> Data Store Write3/1, Mux/1  "HwTqIdptMin"
  Demux/2 -> RngLimMotAgMecIdptSig/1(MotAgMeclIdptSig)  "MotAgMeclIdptSig"

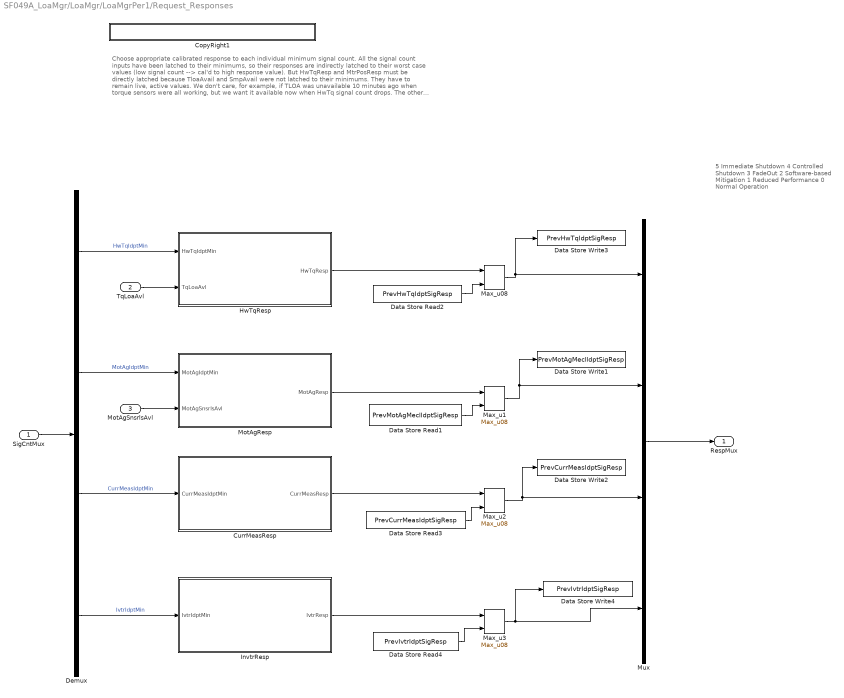
== system SF049A_LoaMgr/LoaMgr/LoaMgrPer1/Request_Responses ==
  note: 5 Immediate Shutdown
      | 4 Controlled Shutdown
      | 3 FadeOut
      | 2 Software-based Mitigation
      | 1 Reduced Performance
      | 0 Normal Operation
  note: Choose appropriate calibrated response to each individual minimum signal count.  All the signal count inputs have been latched to their minimums,
      | so their responses are indirectly latched to their worst case values (low signal count --> cal'd to high response value).  But HwTqResp and
      | MtrPosResp must be directly latched because TloaAvail and SmpAvail were not latched to their minimums.  They have to remain live, active values.
      | We don't care, for example, if TLOA was unavailable 10 minutes ago when torque sensors were all working, but we want it available now when
      | HwTq signal count drops.
      |
      | The other two (MotCurrResp and IvtrResp) are being latched as defensive programming against inappropriate calibration values.  Peer review group
      | had concerns about a scenerio like this:  (IdptSig=2, Resp=Normal) and (IdptSig=1, Resp=SwMtgtn) and (IdptSig=0, Resp=Normal).
  SigCntMux : Inport
  TqLoaAvl : Inport  RequirementInfo={} %GIDa_4b8ec4aa_ba4b_4697_acc3_b1d8ec5a65c5  Port=2
  MotAgSnsrlsAvl : Inport  RequirementInfo={} %GIDa_a180ff54_fcb3_4e7d_9f19_d2f4d86e150e  Port=3
  CopyRight1 : Subsystem  Description=|  mask(Copyright Information){none=on}
      | Copyright info block.                                               
      |                                                                     
      | Place copyright information at the top of every subsystem in design.
      mask prompts: none "No parameters"
      mask help: Place copyright information at the top of every subsystem in design.
      mask Display:
      | NxtrConf = 'Nexteer Confidential';
      | 
      | sys = bdroot; %handle for the current model ("system")
      | first = get_param(sys,'Created');
      | first = first(end-3:end);  %year is last four digits
      | 
      | last = get_param(sys,'LastModifiedDate');
      | if isempty(last)
      |     last = datestr(now,'yyyy');
      | else
      |     last = last(end-3:end);
      | end
      | 
      | if strcmp(first,last)
      |     fprintf('%s -- Copyright %s Nexteer',NxtrConf,first)
      | else
      |     fprintf('%s -- %s%s- %s Nexteer',NxtrConf,char(169),first,last)
      | end
  CurrMeasResp : Subsystem
  Data Store Read1 : DataStoreRead  RequirementInfo="{'linktype_rmi_doors' '00012fd5 (/E-STEER Core/SubSystem Specifications/Application Functions - EA4/SF049A Loss of Assist Manager)' '#SF049A_125' 'true' 'REQ:  SF049A_125' '' } %GIDa_389f8ad6_9e40_4a83_b6dd_445c5853b25a"  DataStoreName=PrevMotAgMeclIdptSigResp
  Data Store Read2 : DataStoreRead  RequirementInfo="{'linktype_rmi_doors' '00012fd5 (/E-STEER Core/SubSystem Specifications/Application Functions - EA4/SF049A Loss of Assist Manager)' '#SF049A_122' 'true' 'REQ:  SF049A_122' '' } %GIDa_bb75ec4f_3d69_4faf_b14f_32a1ba9c590e"  DataStoreName=PrevHwTqIdptSigResp
  Data Store Read3 : DataStoreRead  RequirementInfo="{'linktype_rmi_doors' '00012fd5 (/E-STEER Core/SubSystem Specifications/Application Functions - EA4/SF049A Loss of Assist Manager)' '#SF049A_127' 'true' 'REQ:  SF049A_127' '' } %GIDa_09473033_6a26_4fdd_9846_9289b114c28e"  DataStoreName=PrevCurrMeasIdptSigResp
  Data Store Read4 : DataStoreRead  RequirementInfo="{'linktype_rmi_doors' '00012fd5 (/E-STEER Core/SubSystem Specifications/Application Functions - EA4/SF049A Loss of Assist Manager)' '#SF049A_129' 'true' 'REQ:  SF049A_129' '' } %GIDa_e0a242fc_43c8_4993_9f82_37b86aa31e46"  DataStoreName=PrevIvtrIdptSigResp
  Data Store Write1 : DataStoreWrite  RequirementInfo="{'linktype_rmi_doors' '00012fd5 (/E-STEER Core/SubSystem Specifications/Application Functions - EA4/SF049A Loss of Assist Manager)' '#SF049A_125' 'true' 'REQ:  SF049A_125' '' } %GIDa_7401fc51_171e_46ae_8be9_1ad2cf9f29c6"  DataStoreName=PrevMotAgMeclIdptSigResp
  Data Store Write2 : DataStoreWrite  RequirementInfo="{'linktype_rmi_doors' '00012fd5 (/E-STEER Core/SubSystem Specifications/Application Functions - EA4/SF049A Loss of Assist Manager)' '#SF049A_127' 'true' 'REQ:  SF049A_127' '' } %GIDa_8f3213c6_02a7_48d7_9a78_ca94d3a67fa7"  DataStoreName=PrevCurrMeasIdptSigResp
  Data Store Write3 : DataStoreWrite  RequirementInfo="{'linktype_rmi_doors' '00012fd5 (/E-STEER Core/SubSystem Specifications/Application Functions - EA4/SF049A Loss of Assist Manager)' '#SF049A_122' 'true' 'REQ:  SF049A_122' '' } %GIDa_39fa06ce_f06b_4a8e_aa84_ee71d1f5dd7f"  DataStoreName=PrevHwTqIdptSigResp
  Data Store Write4 : DataStoreWrite  RequirementInfo="{'linktype_rmi_doors' '00012fd5 (/E-STEER Core/SubSystem Specifications/Application Functions - EA4/SF049A Loss of Assist Manager)' '#SF049A_129' 'true' 'REQ:  SF049A_129' '' } %GIDa_8d6d1a61_df4d_4174_89de_4d81c6eed90c"  DataStoreName=PrevIvtrIdptSigResp
  Demux : Demux
  HwTqResp : Subsystem
  InvtrResp : Subsystem
  Max_u08 : NxtrMax/Max_u08  RequirementInfo="{'linktype_rmi_doors' '00012fd5 (/E-STEER Core/SubSystem Specifications/Application Functions - EA4/SF049A Loss of Assist Manager)' '#SF049A_122' 'true' 'REQ:  SF049A_122' '' } %GIDa_def3381f_7095_4b8f_8f45_3e005c8a337c"  SFunctionSpec="uint8 y1 = Max_u08( uint8 u1,  uint8 u2)"
      settings: AttributesFormatString=%<Name>
  Max_u1 : NxtrMax/Max_u08  RequirementInfo="{'linktype_rmi_doors' '00012fd5 (/E-STEER Core/SubSystem Specifications/Application Functions - EA4/SF049A Loss of Assist Manager)' '#SF049A_125' 'true' 'REQ:  SF049A_125' '' } %GIDa_87874c5c_6402_49e7_af06_e4a0dcdbd806"  SFunctionSpec="uint8 y1 = Max_u08( uint8 u1,  uint8 u2)"
      settings: AttributesFormatString=%<Name>
  Max_u2 : NxtrMax/Max_u08  RequirementInfo="{'linktype_rmi_doors' '00012fd5 (/E-STEER Core/SubSystem Specifications/Application Functions - EA4/SF049A Loss of Assist Manager)' '#SF049A_127' 'true' 'REQ:  SF049A_127' '' } %GIDa_89d9503c_e674_41f1_813d_48b716d0c972"  SFunctionSpec="uint8 y1 = Max_u08( uint8 u1,  uint8 u2)"
      settings: AttributesFormatString=%<Name>
  Max_u3 : NxtrMax/Max_u08  RequirementInfo="{'linktype_rmi_doors' '00012fd5 (/E-STEER Core/SubSystem Specifications/Application Functions - EA4/SF049A Loss of Assist Manager)' '#SF049A_129' 'true' 'REQ:  SF049A_129' '' } %GIDa_cec7e86e_dd6f_45cf_b92b_441172dbf754"  SFunctionSpec="uint8 y1 = Max_u08( uint8 u1,  uint8 u2)"
      settings: AttributesFormatString=%<Name>
  MotAgResp : Subsystem
  Mux : Mux
  RespMux : Outport
  wires:
  Data Store Read4/1 -> Max_u3/2
  Data Store Read3/1 -> Max_u2/2
  Data Store Read1/1 -> Max_u1/2
  Max_u1/1 -> Mux/2, Data Store Write1/1
  Data Store Read2/1 -> Max_u08/2
  Max_u3/1 -> Mux/4, Data Store Write4/1
  InvtrResp/1(IvtrResp) -> Max_u3/1
  Max_u2/1 -> Mux/3, Data Store Write2/1
  CurrMeasResp/1(CurrMeasResp) -> Max_u2/1
  MotAgResp/1(MotAgResp) -> Max_u1/1
  Max_u08/1 -> Mux/1, Data Store Write3/1
  HwTqResp/1(HwTqResp) -> Max_u08/1
  MotAgSnsrlsAvl/1 -> MotAgResp/2(MotAgSnsrlsAvl)
  TqLoaAvl/1 -> HwTqResp/2(TqLoaAvl)
  Mux/1 -> RespMux/1
  SigCntMux/1 -> Demux/1
  Demux/2 -> MotAgResp/1(MotAgIdptMin)  "MotAgIdptMin"
  Demux/4 -> InvtrResp/1(IvtrIdptMin)  "IvtrIdptMin"
  Demux/3 -> CurrMeasResp/1(CurrMeasIdptMin)  "CurrMeasIdptMin"
  Demux/1 -> HwTqResp/1(HwTqIdptMin)  "HwTqIdptMin"
